simulink model "examen"  (R2018b)
settings: Solver=ode1  StartTime=0.0  StopTime=20  FixedStep=.001  RelTol=1e-3
values from neighbouring files (symbols this model uses):
  A2 = [0  1  0; 0  0  1; -6732  788  -5]    [matlab.mat]
  A3 = [0  1  0; 0  0  1; 1683  788  -5]    [matlab.mat]    (also in problema3.m = [0 1 0; 0 0 1;1683 788 -5])
  A6 = [0  1  0; 0  0  1; -9  27  -11]    [matlab.mat]    (also in problema6.m = [0 1 0; 0 0 1;-9 27 -11])
  A9 = [0  1  0; 0  0  1; 1683  -439  37]    [matlab.mat]    (also in problema4.m = [0 1 0; 0 0 1;1683 -439 37])
  B2 = [0 0 1]    [matlab.mat]
  B3 = [0 0 1]    [matlab.mat]    (also in problema3.m = [0 0 1]')
  B6 = [0 0 1]    [matlab.mat]    (also in problema6.m = [0 0 1]')
  B9 = [0 0 1]    [matlab.mat]    (also in problema4.m = [0 0 1]')
  C2 = [2 5 0]    [matlab.mat]
  C3 = [9 7 0]    [matlab.mat]    (also in problema3.m)
  C6 = [1 0 0]    [matlab.mat]    (also in problema6.m)
  C9 = [1 0 0]    [matlab.mat]    (also in problema4.m)
  K2 = [-6716 799 1]    [matlab.mat]
  K3 = [1689 799 1]    [matlab.mat]
  K9 = [1689 -428 43]    [matlab.mat]    (also in problema4.m = acker(A9,B9,[-1,-2,-3]))
  L9 = [70 2513 65254]    [matlab.mat]    (also in problema4.m = acker(A9',C9',[-10 -11 -12])')
libraries: cstblocks x2
settings Model: Creator=Abraham Pérez  LastModifiedBy=Abraham Pérez
settings SolverCC: InitialStep=.001

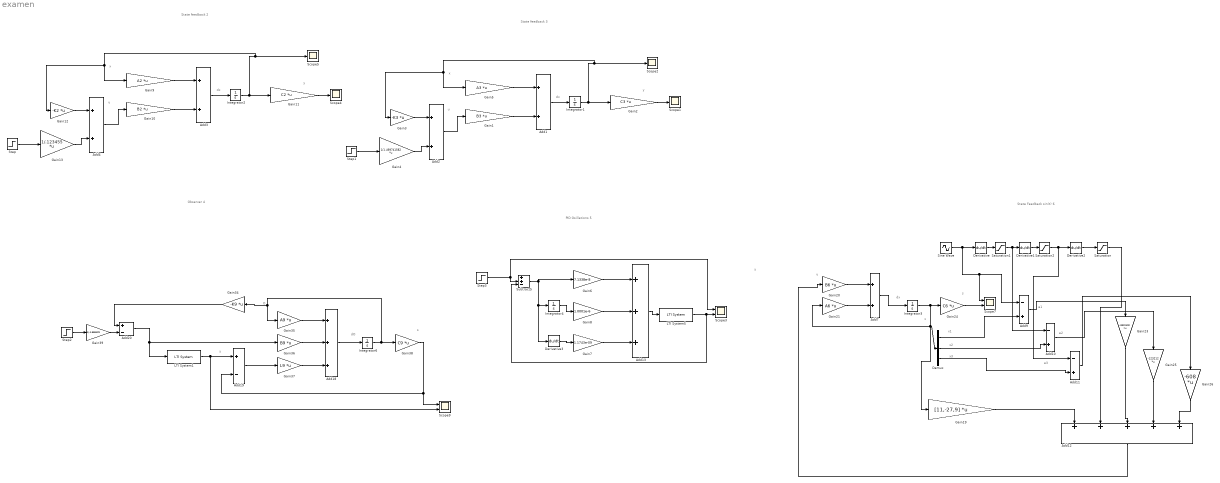
== system examen ==
  note: State feedback 2
  note: dx
  note: x
  note: y
  note: u
  note: y
  note: u
  note: State feedback 3
  note: dx
  note: x
  note: y
  note: Observer 4
  note: x1
  note: x
  note: e3
  note: s
  note: x3
  note: x2
  note: u
  note: dx
  note: e2
  note: State Feedback sin(t) 6
  note: e1
  note: PID Osillations 5
  note: dO
  note: s
  note: O
  note: y
  Add{1..4,7} (5 alike) : Sum
  Add10 : Sum  Inputs=-+
  Add11 : Sum  Inputs=-+
  Add12 : Sum  Inputs=+++++
  Add13 : Sum  Inputs=+++
  Add18 : Sum  Inputs=+++
  Add19 : Sum  Inputs=+-
  Add20 : Sum  Inputs=+-
  Add9 : Sum  Inputs=-+
  Demux : Demux  Outputs=3
  Derivative{,1..3} (4 alike) : Derivative
  Gain1 : Gain  Gain=B3  Multiplication=Matrix(K*u)
  Gain10 : Gain  Gain=B2  Multiplication=Matrix(K*u)
  Gain11 : Gain  Gain=C2  Multiplication=Matrix(K*u)
  Gain12 : Gain  Gain=-K2  Multiplication=Matrix(K*u)
  Gain13 : Gain  Gain=1/.123455  Multiplication=Matrix(K*u)
  Gain19 : Gain  Gain=[11,-27,9]  Multiplication=Matrix(K*u)
  Gain2 : Gain  Gain=C3  Multiplication=Matrix(K*u)
  Gain20 : Gain  Gain=B6  Multiplication=Matrix(K*u)
  Gain21 : Gain  Gain=A6  Multiplication=Matrix(K*u)
  Gain23 : Gain  Gain=-8322400  Multiplication=Matrix(K*u)
  Gain24 : Gain  Gain=C6  Multiplication=Matrix(K*u)
  Gain25 : Gain  Gain=-123212  Multiplication=Matrix(K*u)
  Gain26 : Gain  Gain=-608  Multiplication=Matrix(K*u)
  Gain3 : Gain  Gain=-K3  Multiplication=Matrix(K*u)
  Gain34 : Gain  Gain=-K9  Multiplication=Matrix(K*u)
  Gain35 : Gain  Gain=A9  Multiplication=Matrix(K*u)
  Gain36 : Gain  Gain=B9  Multiplication=Matrix(K*u)
  Gain37 : Gain  Gain=L9  Multiplication=Matrix(K*u)
  Gain38 : Gain  Gain=C9  Multiplication=Matrix(K*u)
  Gain39 : Gain  Gain=1/-1.668429
  Gain4 : Gain  Gain=1/1.499741582  Multiplication=Matrix(K*u)
  Gain5 : Gain  Gain=A3  Multiplication=Matrix(K*u)
  Gain6 : Gain  Gain=7.1338e-8
  Gain7 : Gain  Gain=1.1743e-09
  Gain8 : Gain  Gain=1.0001e-6
  Gain9 : Gain  Gain=A2  Multiplication=Matrix(K*u)
  Integrator1 : Integrator  InitialCondition=[-1 .5 .5 ]
  Integrator2 : Integrator  InitialCondition=[-1 .5 .5 ]
  Integrator3 : Integrator  InitialCondition=[1 0 -1]
  Integrator4 : Integrator
  Integrator6 : Integrator  InitialCondition=[1 0 -1]
  LTI System1 : cstblocks/LTI System  sys=G9  IC=[]
  LTI System5 : cstblocks/LTI System  sys=g5  IC=[]
  Saturation : Saturate  UpperLimit=1  LowerLimit=-1
  Saturation1 : Saturate  UpperLimit=1  LowerLimit=-1
  Saturation2 : Saturate  UpperLimit=1  LowerLimit=-1
  Scope{1..2,4..5} (4 alike) : Scope
  Scope3 : Scope  NumInputPorts=2
  Scope7 : Scope  NumInputPorts=2
  Scope9 : Scope  NumInputPorts=2
  Sine Wave : Sin  Amplitude=17/9  SampleTime=0
  Step : Step  SampleTime=0
  Step1 : Step  After=2  SampleTime=0
  Step2 : Step  After=10  SampleTime=0
  Step3 : Step  After=10  SampleTime=0
  Subtract5 : Sum  Inputs=++-
  wires:
  Step/1 -> Gain13/1
  Gain12/1 -> Add4/1
  Gain13/1 -> Add4/2
  Add4/1 -> Gain10/1
  Gain10/1 -> Add3/2
  Gain11/1 -> Scope4/1
  Gain9/1 -> Add3/1
  Add3/1 -> Integrator2/1
  Integrator2/1 -> Gain11/1, Scope5/1, Gain9/1, Gain12/1
  Step1/1 -> Gain4/1
  Add2/1 -> Gain1/1
  Integrator1/1 -> Gain2/1, Scope2/1, Gain5/1, Gain3/1
  Gain5/1 -> Add1/1
  Gain2/1 -> Scope1/1
  Add1/1 -> Integrator1/1
  Gain1/1 -> Add1/2
  Gain4/1 -> Add2/2
  Gain3/1 -> Add2/1
  Saturation/1 -> Add12/2
  Add11/1 -> Gain26/1
  Saturation2/1 -> Add11/1, Derivative2/1
  Gain19/1 -> Add12/1
  Derivative2/1 -> Saturation/1
  Gain26/1 -> Add12/5
  Demux/3 -> Add11/2
  Add12/1 -> Gain20/1
  Gain25/1 -> Add12/4
  Demux/2 -> Add10/2
  Gain23/1 -> Add12/3
  Integrator3/1 -> Gain19/1, Gain21/1, Demux/1, Gain24/1
  Gain20/1 -> Add7/1
  Gain24/1 -> Scope7/2
  Add7/1 -> Integrator3/1
  Gain21/1 -> Add7/2
  Derivative1/1 -> Saturation2/1
  Add10/1 -> Gain25/1
  Add9/1 -> Gain23/1
  Demux/1 -> Add9/2
  Saturation1/1 -> Add10/1, Derivative1/1
  Derivative/1 -> Saturation1/1
  Sine Wave/1 -> Scope7/1, Add9/1, Derivative/1
  Derivative3/1 -> Gain7/1
  Integrator4/1 -> Gain8/1
  Gain7/1 -> Add13/3
  Step3/1 -> Scope3/1, Subtract5/2
  Gain8/1 -> Add13/2
  LTI System5/1 -> Scope3/2, Subtract5/3
  Gain6/1 -> Add13/1
  Subtract5/1 -> Derivative3/1, Integrator4/1, Gain6/1
  Add13/1 -> LTI System5/1
  Gain34/1 -> Add20/1
  Gain36/1 -> Add18/2
  LTI System1/1 -> Scope9/2, Add19/1
  Integrator6/1 -> Gain38/1, Gain35/1, Gain34/1
  Add20/1 -> Gain36/1, LTI System1/1
  Gain38/1 -> Scope9/1, Add19/2
  Gain35/1 -> Add18/1
  Gain37/1 -> Add18/3
  Step2/1 -> Gain39/1
  Gain39/1 -> Add20/2
  Add19/1 -> Gain37/1
  Add18/1 -> Integrator6/1
